simulink model "Model_SimulinkTemplate"  (R2020b)
settings: Solver=ode23tb  StartTime=0.0  StopTime=10.0  RelTol=1e-3
settings Model: Creator=prenk  LastModifiedBy=renkert2

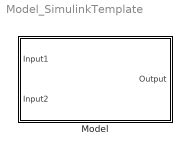
== system Model_SimulinkTemplate ==
  Model : Subsystem  mask{x_0=0}

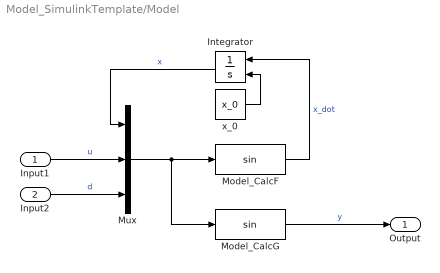
== system Model_SimulinkTemplate/Model ==
  Input1 : Inport
  Input2 : Inport  Port=2
  Integrator : Integrator  InitialConditionSource=external
  Model_CalcF : MATLABFcn
  Model_CalcG : MATLABFcn
  Mux : Mux  Inputs=3
  x_0 : Constant  Value=x_0  VectorParams1D=off
  Output : Outport
  wires:
  Model_CalcF/1 -> Integrator/1  "x_dot"
  Input1/1 -> Mux/2  "u"
  Model_CalcG/1 -> Output/1  "y"
  x_0/1 -> Integrator/2
  Input2/1 -> Mux/3  "d"
  Integrator/1 -> Mux/1  "x"
  Mux/1 -> Model_CalcG/1, Model_CalcF/1
